simulink library "tqd"  (R2021b)
settings: Solver=VariableStepAuto  StartTime=0.0  StopTime=10.0  RelTol=1e-3
undefined symbols (not defined in the file): ATQD_AfterTqMinGain_X_Deg, ATQD_APSCreepBaseTqD_X_kph, ATQD_APSCreepBaseTqD_Y_Deg, ATQD_APSCreepBaseTqR_X_kph, ATQD_APSCreepBaseTqR_Y_Deg, ATQD_APSCreepIterm_X_kph, ATQD_APSCreepIterm_Y_kph, ATQD_APSCreepPterm_X_kph, ATQD_APSCreepPterm_Y_kph, ATQD_APSDecReq_X_kph, ATQD_APSDecReq_Y_mps2, ATQD_APSDecReqCMD_X_kph, ATQD_APSDecReqTs_X_pct, ATQD_APSDecTimeGain_X_Deg, ATQD_APSDecTimeGain_Y_s, ATQD_APSReqLowSpd_X_Deg, ATQD_AutoHoldReleaseBPS_X_Deg, ATQD_AWDLoadTrqnsGain_X_kg, ATQD_AWDLoadTrqnsGain_Y_pct, ATQD_BOSEnBPSPosn_X_kph, ATQD_BOSMap_X_rpm, ATQD_BOSMap_Y_pct, ATQD_CreepBaseTqD_X_kph, ATQD_CreepBaseTqD_Y_Deg, ATQD_CreepBaseTqR_X_kph, ATQD_CreepBaseTqR_Y_Deg, ATQD_CreepBPSDisPosn_X_Deg, ATQD_CreepBPSDisPosnR_X_Deg, ATQD_CreepBPSEnPosn_X_Deg, ATQD_CreepBPSEnPosnR_X_Deg, ATQD_CreepDeltaTq_X_kph, ATQD_CreepIterm_X_kph, ATQD_CreepIterm_Y_kph, ATQD_CreepItermMaxLimit_X_pct, ATQD_CreepPreloadTime_X_kph, ATQD_CreepPreloadTq_X_kph, ATQD_CreepPreloadTq_Y_s, ATQD_CreepProtTq_X_Deg, ATQD_CreepPterm_X_kph, ATQD_CreepPterm_Y_kph, ATQD_CreepRrTqSpRat_X_rpm, ATQD_CreepRrTqSpRat_Y_Nm, ATQD_CreepTargetSpdD_X_pct, ATQD_CreepTargetSpdR_X_pct, ATQD_ECOTqMapD_X_rpm, ATQD_ECOTqMapD_Y_pct, ATQD_EMTqMapD_X_rpm, ATQD_EMTqMapD_Y_pct, ATQD_EOPDTqMapDCon_X_rpm, ATQD_EOPDTqMapDCon_Y_Deg, ATQD_EscapeModePedTq_X_pct, ATQD_EscapeModePedTq_Y_rpm, ATQD_EscapeModePedTqFr_X_pct, ATQD_EscapeModePedTqFr_Y_rpm, ATQD_EstInitVehWeight_X_c, ATQD_FAfterTqCMDGain_X_rpm, ATQD_FAfterTqCMDGain_Y_pct, ATQD_FrLossMAPLowV_X_rpm, ATQD_FrLossMAPLowV_Y_Nm, ATQD_FrMotActReduce_X_rpm ... (+772)
libraries: simulink x211, hcu_lib x179, tqr x3
(part 5 of 28)

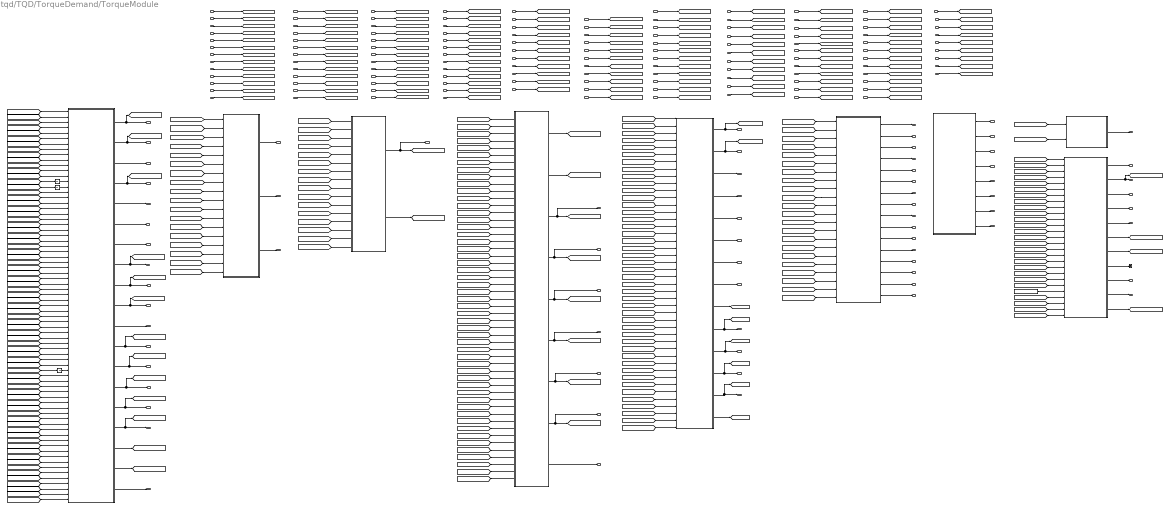
== system tqd/TQD/TorqueDemand/TorqueModule ==
  note: Input Signals
  VTQD_LowIdleAccPedal_flg : Inport
  VPMM_DrivetrainSelect_enum : Inport  Port=2
  VTQD_RollRegenDisableReq_flg : Inport  Port=3
  VTQD_GearActualPosn_enum : Inport  Port=4
  VTQD_CreepON_flg : Inport  Port=5
  VTQD_BrkSwSta_flg : Inport  Port=6
  VTQD_LimpHomeAct_flg : Inport  Port=7
  VTQD_EVDriveMode_enum : Inport  Port=8
  VTQD_RegenMode_enum : Inport  Port=9
  VINP_VehSpeed_kph : Inport  Port=10
  VTQD_TqTargetShaftSpd_rpm : Inport  Port=11
  VTQD_FrShaftSpd_rpm : Inport  Port=12
  VTQD_RrShaftSpd_rpm : Inport  Port=13
  VTQD_ActAPSPosn_pct : Inport  Port=14
  VTQD_ActBPSPosn_pct : Inport  Port=15
  VINP_FrPTCSActive_flg : Inport  Port=16
  VINP_RrPTCSActive_flg : Inport  Port=17
  VINP_FrntAxlTrqReqDrv_Nm : Inport  Port=18
  VINP_RearAxlTrqReqDrv_Nm : Inport  Port=19
  VINP_FrRBCActive_flg : Inport  Port=20
  VINP_RrRBCActive_flg : Inport  Port=21
  VINP_FrntAxlTrqReqBrk_Nm : Inport  Port=22
  VINP_RearAxlTrqReqBrk_Nm : Inport  Port=23
  VVMC_ADASActive_flg : Inport  Port=24
  VVMC_ADASWhlTqReq_Nm : Inport  Port=25
  VVMC_CruzActive_flg : Inport  Port=26
  VVMC_CruzWhlTqReq_Nm : Inport  Port=27
  VVMC_MSAActive_flg : Inport  Port=28
  VVMC_MSAWhlTqReq_Nm : Inport  Port=29
  VVMC_APSActive_flg : Inport  Port=30
  VINP_HVBPwrAvailDchrg_kw : Inport  Port=31
  VTQD_EstVehWeightResult_kg : Inport  Port=32
  VVMC_LongAcc_Gps : Inport  Port=33
  VINP_HVBPwrAvailChrg_kw : Inport  Port=34
  VINP_FrRegenAvailTq_Nm : Inport  Port=35
  VINP_RrRegenAvailTq_Nm : Inport  Port=36
  VINP_FrTMSpd_RPM : Inport  Port=37
  VINP_RrTMSpd_RPM : Inport  Port=38
  VINP_FrEDURealTMTq_Nm : Inport  Port=39
  VINP_RrEDURealTMTq_Nm : Inport  Port=40
  VTQD_ParkRequest_flg : Inport  Port=41
  VPMM_PwrSta_enum : Inport  Port=42
  VTQD_MCUReady4Ext_flg : Inport  Port=43
  VINP_HVBattErr_flg : Inport  Port=44
  VINP_DCDCFaultSta_enum : Inport  Port=45
  VINP_ADASForceIdle_flg : Inport  Port=46
  VTQD_TMRotateDirction_enum : Inport  Port=47
  VINP_LongAccel_Gps : Inport  Port=48
  VTQR_ActualFEDUWhlTqReq_Nm : Inport  Port=49
  VTQR_ActualREDUWhlTqReq_Nm : Inport  Port=50
  VINP_BrkPedalPos_pct : Inport  Port=51
  VTQD_RDCActive_enum : Inport  Port=52
  VVMC_ActMaxSlideRate_pct : Inport  Port=53
  VINP_FrMotorAvailTq_Nm : Inport  Port=54
  VINP_RrMotorAvailTq_Nm : Inport  Port=55
  task_time_s : Inport  Port=56
  VINP_HSAActive_flg : Inport  Port=57
  VTQR_NoABSFEDUWhlTqReq_Nm : Inport  Port=58
  VTQR_NoABSREDUWhlTqReq_Nm : Inport  Port=59
  VINP_AVHActive_flg : Inport  Port=60
  VINP_EPBErrSta_enum : Inport  Port=61
  VVMC_APSSpeedCMD_kph : Inport  Port=62
  VVMC_APSReq_enum : Inport  Port=63
  VINP_ACCVehHoldReq_flg : Inport  Port=64
  VTQD_DriveProtRemove_flg : Inport  Port=65
  VVMC_ACCRequiredAccel_mps2 : Inport  Port=66
  VVMC_EstSlope_Deg : Inport  Port=67
  VTQD_SysMode_enum : Inport  Port=68
  VINP_SWCResUpSta_flg : Inport  Port=69
  VINP_DrDoorSW_flg : Inport  Port=70
  VINP_PsDoorSW_flg : Inport  Port=71
  VINP_RRDoorSW_flg : Inport  Port=72
  VINP_RLDoorSW_flg : Inport  Port=73
  VINP_HoodSW_flg : Inport  Port=74
  VINP_TailgateSW_flg : Inport  Port=75
  VINP_ADASACCSta_enum : Inport  Port=76
  VINP_EPBSta_enum : Inport  Port=77
  VVMC_ActLRSlideRate_pct : Inport  Port=78
  VVMC_ActRRSlideRate_pct : Inport  Port=79
  VINP_SASAngle_Deg : Inport  Port=80
  VINP_YawRate_degps : Inport  Port=81
  VVMC_ActStESCYaw_degps : Inport  Port=82
  VVMC_CAASActive_flg : Inport  Port=83
  VINP_HVBattSOC_pct : Inport  Port=84
  VVMC_RearTqRatio_rat : Inport  Port=85
  VINP_ESCActive_flg : Inport  Port=86
  VINP_ABSActive_flg : Inport  Port=87
  VINP_IVISnowModeCmd_flg : Inport  Port=88
  VINP_VehicleType_enum : Inport  Port=89
  VTQD_IVIRockModeEn_flg : Inport  Port=90
  VTQR_RShaftSpdTqLimLow_flg : Inport  Port=91
  VTQR_RTimerTqLimLow_flg : Inport  Port=92
  VTQR_FShaftSpdTqLimLow_flg : Inport  Port=93
  VTQR_FTimerTqLimLow_flg : Inport  Port=94
  VINP_LFRawWhlSpeed_kph : Inport  Port=95
  VINP_LRRawWhlSpeed_kph : Inport  Port=96
  VINP_RFRawWhlSpeed_kph : Inport  Port=97
  VINP_RRRawWhlSpeed_kph : Inport  Port=98
  VTQD_RearSlideRate_pct : Inport  Port=99
  VTQD_FrontSlideRate_pct : Inport  Port=100
  VINP_SWC2RCustomizeSta_flg : Inport  Port=101
  VTQR_FrFirstOrderInpTs_c : Inport  Port=102
  VTQR_RrFirstOrderInpTs_c : Inport  Port=103
  VTQR_FrRateLimitInc_Nm : Inport  Port=104
  VTQR_FrRateLimitDec_Nm : Inport  Port=105
  VTQR_RrRateLimitInc_Nm : Inport  Port=106
  VTQR_RrRateLimitDec_Nm : Inport  Port=107
  VINP_FrMCUDCBusVolt_V : Inport  Port=108
  VINP_RrMCUDCBusVolt_V : Inport  Port=109
  VTQD_ActWhlSkipSta_enum : Inport  Port=110
  VTQD_SkipDirect_enum : Inport  Port=111
  VDDM_EPB1Err_flg : Inport  Port=112
  VDDM_ESC1Err_flg : Inport  Port=113
  VDDM_ESC5Err_flg : Inport  Port=114
  VDDM_EPBSigErrCFS_flg : Inport  Port=115
  VINP_FrMCUTemp_C : Inport  Port=116
  VINP_FrTMTemp_C : Inport  Port=117
  VINP_RrMCUTemp_C : Inport  Port=118
  VINP_RrTMTemp_C : Inport  Port=119
  VINP_ADASAEBSta_enum : Inport  Port=120
  VTQR_FrTqZeroTransLowBound_Nm : Inport  Port=121
  VTQR_RrTqZeroTransUpBound_Nm : Inport  Port=122
  VDDM_VehMalfunLevel_enum : Inport  Port=123
  VDDM_MCUF1Err_flg : Inport  Port=124
  VDDM_MCUR1Err_flg : Inport  Port=125
  VDDM_Shifter1Err_flg : Inport  Port=126
  VDDM_ShifterSigErrCFS_flg : Inport  Port=127
  VDDM_4D2CErr_flg : Inport  Port=128
  VDDM_RegenErrCFS_flg : Inport  Port=129
  VDDM_VCURAPSErrLv2_flg : Inport  Port=130
  AvaliableTqLimit : Subsystem  AncestorBlock=tqd0/TQD/TorqueDemand/TorqueModule/AvaliableTqLimit
  Constant34 : Constant  Value=KTQD_IVICreepOnSW_flg
  DriverWhlTqDem : Subsystem
  ExtTqFuncHandShaking : Subsystem
  OPD Hold : Subsystem
  Signal for ESC : Subsystem  AncestorBlock=tqd0/TQD/TorqueDemand/TorqueModule/Signal for ESC
  Signals for BCM : Subsystem
  Signals for MCU : Subsystem
  Terminator : Terminator
  TqCoordination : Subsystem
  TqDistribution : Subsystem  AncestorBlock=tqd0/TQD/TorqueDemand/TorqueModule/TqDistribution
  Unit Delay : UnitDelay  SampleTime=-1  HasFrameUpgradeWarning=on
  Unit Delay1 : UnitDelay  SampleTime=-1  HasFrameUpgradeWarning=on
  Unit Delay2 : UnitDelay  SampleTime=-1  HasFrameUpgradeWarning=on
  VTQD_DriverWhlTqDem_Nm : Outport
  VTQD_TqSourceFr_enum : Outport  Port=2
  VTQD_TqSourceRr_enum : Outport  Port=3
  VTQD_RollRegenEnable_flg : Outport  Port=4
  VTQD_EVDriveModeValid_flg : Outport  Port=5
  VTQD_AfterAvailableTqDemFr_Nm : Outport  Port=6
  VTQD_AfterAvailableTqDemRr_Nm : Outport  Port=7
  VTQD_FrEDUAvailBrkRgnTq_Nm : Outport  Port=8
  VTQD_RrEDUAvailBrkRgnTq_Nm : Outport  Port=9
  VTQD_FrRgnDecrSta_flg : Outport  Port=10
  VTQD_RrRgnDecrSta_flg : Outport  Port=11
  VTQD_FrEDUActTq_Nm : Outport  Port=12
  VTQD_RrEDUActTq_Nm : Outport  Port=13
  VTQD_FrEDURolRgnTq_Nm : Outport  Port=14
  VTQD_RrEDURolRgnTq_Nm : Outport  Port=15
  VTQD_FrEDUSpd_rpm : Outport  Port=16
  VTQD_RrEDUSpd_rpm : Outport  Port=17
  VTQD_FrEDUSpdValid_flg : Outport  Port=18
  VTQD_FrEDUActTqValid_flg : Outport  Port=19
  VTQD_FrEDURolRgnTqValid_flg : Outport  Port=20
  VTQD_FrEDUAvailBrkRgnTqV_flg : Outport  Port=21
  VTQD_RrEDUSpdValid_flg : Outport  Port=22
  VTQD_RrEDUActTqValid_flg : Outport  Port=23
  VTQD_RrEDURolRgnTqValid_flg : Outport  Port=24
  VTQD_RrEDUAvailBrkRgnTqV_flg : Outport  Port=25
  VTQD_RgnAbnorSta_flg : Outport  Port=26
  VTQD_PTCSPermSta_flg : Outport  Port=27
  VTQD_FrRgnPermSta_flg : Outport  Port=28
  VTQD_RrRgnPermSta_flg : Outport  Port=29
  VTQD_DriverWhlTqDemFr_Nm : Outport  Port=30
  VTQD_DriverWhlTqDemRr_Nm : Outport  Port=31
  VTQD_ExternalTqAllow_flg : Outport  Port=32
  VTQD_FrIdcMin_A : Outport  Port=33
  VTQD_FrIdcMax_A : Outport  Port=34
  VTQD_FrUdcMin_V : Outport  Port=35
  VTQD_FrUdcMax_V : Outport  Port=36
  VTQD_RrIdcMin_A : Outport  Port=37
  VTQD_RrIdcMax_A : Outport  Port=38
  VTQD_RrUdcMin_V : Outport  Port=39
  VTQD_RrUdcMax_V : Outport  Port=40
  VTQD_CoordWhlTqDemFr_Nm : Outport  Port=41
  VTQD_CoordWhlTqDemRr_Nm : Outport  Port=42
  VTQD_CreepEnable_flg : Outport  Port=43
  VTQD_ReBrakeLPReq_flg : Outport  Port=44
  VTQD_LoSpdBrkCtrl_flg : Outport  Port=45
  VTQD_BOSEnable_flg : Outport  Port=46
  VTQD_ExtShftAllow_flg : Outport  Port=47
  VTQD_OPDOn2Off_flg : Outport  Port=48
  VTQD_PreLoadHold_flg : Outport  Port=49
  VTQD_PreLoadPreEn_flg : Outport  Port=50
  VTQD_CreepPrLoadEnable_flg : Outport  Port=51
  VTQD_APSStaSys_enum : Outport  Port=52
  VTQD_APSReq_enum : Outport  Port=53
  VTQD_APSDecReqA_flg : Outport  Port=54
  VTQD_APSDecReq_mps2 : Outport  Port=55
  VTQD_ActParkRequest_flg : Outport  Port=56
  VTQD_RegenTqLimitEn_flg : Outport  Port=57
  VTQD_ExtDoorAllow_flg : Outport  Port=58
  VTQD_WhlTqCapGenFr_Nm : Outport  Port=59
  VTQD_WhlTqCapGenRr_Nm : Outport  Port=60
  VTQD_OPDHoldAllowPark_flg : Outport  Port=61
  VTQD_OPDHoldLamp_flg : Outport  Port=62
  VTQD_CreepBaseTqD_Nm : Outport  Port=63
  VTQD_VehActSpd_kph : Outport  Port=64
  VTQD_CoordTqDem_Nm : Outport  Port=65
  VTQD_PedAccTqEn_flg : Outport  Port=66
  VTQD_WhlTqCapMotFr_Nm : Outport  Port=67
  VTQD_WhlTqCapMotRr_Nm : Outport  Port=68
  VTQD_CreepTCSActive_flg : Outport  Port=69
  VTQD_EscapModeTqLim_flg : Outport  Port=70
  VTQD_TMEnOutpTqSta_enum : Outport  Port=71
  VTQD_SlideRegenLimTq_Nm : Outport  Port=72
  wires:
  VTQD_ActAPSPosn_pct/1 -> [VTQD_ActAPSPosn_pct]
  VTQD_GearActualPosn_enum/1 -> [VTQD_GearActualPosn_enum]
  VINP_VehSpeed_kph/1 -> [VINP_VehSpeed_kph]
  VTQD_BrkSwSta_flg/1 -> [VTQD_BrkSwSta_flg]
  VTQD_RegenMode_enum/1 -> [VTQD_RegenMode_enum]
  VINP_FrntAxlTrqReqDrv_Nm/1 -> [VINP_FrntAxlTrqReqDrv_Nm]
  VINP_RearAxlTrqReqDrv_Nm/1 -> [VINP_RearAxlTrqReqDrv_Nm]
  VINP_FrPTCSActive_flg/1 -> [VINP_FrPTCSActive_flg]
  VINP_FrntAxlTrqReqBrk_Nm/1 -> [VINP_FrntAxlTrqReqBrk_Nm]
  VINP_RearAxlTrqReqBrk_Nm/1 -> [VINP_RearAxlTrqReqBrk_Nm]
  VTQD_RollRegenDisableReq_flg/1 -> [VTQD_RollRegenDisableReq_flg]
  VINP_FrRBCActive_flg/1 -> [VINP_FrRBCActive_flg]
  VTQD_ActBPSPosn_pct/1 -> [VTQD_ActBPSPosn_pct]
  VVMC_CruzWhlTqReq_Nm/1 -> [VVMC_CruzWhlTqReq_Nm]
  VVMC_CruzActive_flg/1 -> [VVMC_CruzActive_flg]
  VTQD_EVDriveMode_enum/1 -> [VTQD_EVDriveMode_enum]
  VTQD_LimpHomeAct_flg/1 -> [VTQD_LimpHomeAct_flg]
  VTQD_CreepON_flg/1 -> [VTQD_CreepON_flg]
  VTQD_TqTargetShaftSpd_rpm/1 -> [VTQD_TqTargetShaftSpd_rpm]
  VPMM_DrivetrainSelect_enum/1 -> [VPMM_DrivetrainSelect_enum]
  [VTQD_TqTargetShaftSpd_rpm] -> DriverWhlTqDem/10(VTQD_TqTargetShaftSpd_rpm)
  [VTQD_LimpHomeAct_flg] -> DriverWhlTqDem/6(VTQD_LimpHomeAct_flg)
  [VTQD_EVDriveMode_enum] -> DriverWhlTqDem/7(VTQD_EVDriveMode_enum)
  [VTQD_RegenMode_enum] -> DriverWhlTqDem/8(VTQD_RegenMode_enum)
  [VTQD_CreepON_flg] -> DriverWhlTqDem/4("VTQD_CreepON_flg ")
  [VTQD_GearActualPosn_enum] -> DriverWhlTqDem/3(VTQD_GearActualPosn_enum)
  [VTQD_LowIdleAccPedal_flg] -> DriverWhlTqDem/1(VDHP_LowIdleAccPedal_flg)
  [VTQD_ActAPSPosn_pct] -> DriverWhlTqDem/11(VTQD_ActAPSPosn_pct)
  TqDistribution/2(VTQD_RrEDUSpRat_rat) -> [VTQD_RrEDUSpRat_rat]
  TqDistribution/1(VTQD_FrEDUSpRat_rat) -> [VTQD_FrEDUSpRat_rat]
  VINP_HVBPwrAvailChrg_kw/1 -> [VINP_HVBPwrAvailChrg_kw]
  VINP_HVBPwrAvailDchrg_kw/1 -> [VINP_HVBPwrAvailDchrg_kw]
  DriverWhlTqDem/1(VTQD_DriverWhlTqDem_Nm) -> [VTQD_DriverWhlTqDem_Nm], VTQD_DriverWhlTqDem_Nm/1
  [VPMM_DrivetrainSelect_enum] -> TqDistribution/1(VPMM_DrivetrainSelect_enum)
  VVMC_MSAActive_flg/1 -> [VVMC_MSAActive_flg]
  VVMC_MSAWhlTqReq_Nm/1 -> [VVMC_MSAWhlTqReq_Nm]
  VVMC_APSActive_flg/1 -> [VVMC_APSActive_flg]
  VVMC_ADASActive_flg/1 -> [VVMC_ADASActive_flg]
  VVMC_ADASWhlTqReq_Nm/1 -> [VVMC_ADASWhlTqReq_Nm]
  [VTQD_BrkSwSta_flg] -> DriverWhlTqDem/5(VTQD_BrkSwSta_flg)
  [VTQD_ActBPSPosn_pct] -> DriverWhlTqDem/12(VTQD_ActBPSPosn_pct)
  [VINP_VehSpeed_kph] -> DriverWhlTqDem/9(VINP_VehSpeed_kph)
  [VTQD_RollRegenDisableReq_flg] -> DriverWhlTqDem/2(VTQD_RollRegenDisableReq_flg)
  VTQD_FrShaftSpd_rpm/1 -> [VTQD_FrShaftSpd_rpm]
  VTQD_RrShaftSpd_rpm/1 -> [VTQD_RrShaftSpd_rpm]
  VTQD_LowIdleAccPedal_flg/1 -> [VTQD_LowIdleAccPedal_flg]
  DriverWhlTqDem/2(VTQD_RollRegenEnable_flg) -> VTQD_RollRegenEnable_flg/1, [VTQD_RollRegenEnable_flg]
  DriverWhlTqDem/3(VTQD_EVDriveModeValid_flg) -> VTQD_EVDriveModeValid_flg/1
  VINP_RrPTCSActive_flg/1 -> [VINP_RrPTCSActive_flg]
  VINP_RrRBCActive_flg/1 -> [VINP_RrRBCActive_flg]
  VINP_RrTMSpd_RPM/1 -> [VINP_RrTMSpd_rpm]
  VINP_FrTMSpd_RPM/1 -> [VINP_FrTMSpd_rpm]
  VINP_RrRegenAvailTq_Nm/1 -> [VINP_RrRegenAvailTq_Nm]
  VINP_FrRegenAvailTq_Nm/1 -> [VINP_FrRegenAvailTq_Nm]
  VINP_RrEDURealTMTq_Nm/1 -> [VINP_RrEDURealTMTq_Nm]
  VINP_FrEDURealTMTq_Nm/1 -> [VINP_FrEDURealTMTq_Nm]
  AvaliableTqLimit/8(VTQD_RrRgnPermSta_flg) -> VTQD_RrRgnPermSta_flg/1  "VTQD_RrRgnPermSta_flg"
  AvaliableTqLimit/6(VTQD_RrRgnDecrSta_flg) -> VTQD_RrRgnDecrSta_flg/1  "VTQD_RrRgnDecrSta_flg"
  AvaliableTqLimit/7(VTQD_FrRgnPermSta_flg) -> VTQD_FrRgnPermSta_flg/1  "VTQD_FrRgnPermSta_flg"
  [VTQD_RrShaftSpd_rpm] -> AvaliableTqLimit/2(VTQD_RrShaftSpd_rpm)
  [VTQD_FrShaftSpd_rpm] -> AvaliableTqLimit/1(VTQD_FrShaftSpd_rpm)
  AvaliableTqLimit/1(VTQD_AfterAvailableTqDemFr_Nm) -> [VTQD_AfterAvailableTqDemFr_Nm], VTQD_AfterAvailableTqDemFr_Nm/1
  AvaliableTqLimit/5(VTQD_FrRgnDecrSta_flg) -> VTQD_FrRgnDecrSta_flg/1  "VTQD_FrRgnDecrSta_flg"
  AvaliableTqLimit/2(VTQD_AfterAvailableTqDemRr_Nm) -> [VTQD_AfterAvailableTqDemRr_Nm], VTQD_AfterAvailableTqDemRr_Nm/1
  AvaliableTqLimit/3(VTQD_FrEDUAvailBrkRgnTq_Nm) -> VTQD_FrEDUAvailBrkRgnTq_Nm/1
  AvaliableTqLimit/4(VTQD_RrEDUAvailBrkRgnTq_Nm) -> VTQD_RrEDUAvailBrkRgnTq_Nm/1
  [VINP_DCDCFaultSta_enum] -> ExtTqFuncHandShaking/4(VINP_DCDCFaultSta_enum)
  [VINP_HVBattErr_flg] -> ExtTqFuncHandShaking/3(VINP_HVBattErr_flg)
  [VTQD_MCUReady4Ext_flg] -> ExtTqFuncHandShaking/2(VTQD_MCUReady4Ext_flg)
  [VPMM_PwrSta_enum] -> ExtTqFuncHandShaking/1(VPMM_PwrSta_enum)
  VINP_HVBattErr_flg/1 -> [VINP_HVBattErr_flg]
  VINP_ADASForceIdle_flg/1 -> [VINP_ADASForceIdle_flg]
  VTQD_MCUReady4Ext_flg/1 -> [VTQD_MCUReady4Ext_flg]
  VPMM_PwrSta_enum/1 -> [VPMM_PwrSta_enum]
  VINP_DCDCFaultSta_enum/1 -> [VINP_DCDCFaultSta_enum]
  ExtTqFuncHandShaking/1(VTQD_ExternalTqAllow_flg) -> VTQD_ExternalTqAllow_flg/1
  VTQD_TMRotateDirction_enum/1 -> [VTQD_TMRotateDirction_enum]
  [VTQD_TMRotateDirction_enum] -> DriverWhlTqDem/13(VTQD_TMRotateDirction_enum)
  Signals for MCU/8(VTQD_RrUdcMax_V) -> VTQD_RrUdcMax_V/1
  Signals for MCU/5(VTQD_RrIdcMin_A) -> VTQD_RrIdcMin_A/1
  Signals for MCU/3(VTQD_FrUdcMin_V) -> VTQD_FrUdcMin_V/1
  Signals for MCU/2(VTQD_FrIdcMax_A) -> VTQD_FrIdcMax_A/1
  Signals for MCU/7(VTQD_RrUdcMin_V) -> VTQD_RrUdcMin_V/1
  Signals for MCU/6(VTQD_RrIdcMax_A) -> VTQD_RrIdcMax_A/1
  Signals for MCU/4(VTQD_FrUdcMax_V) -> VTQD_FrUdcMax_V/1
  Signals for MCU/1(VTQD_FrIdcMin_A) -> VTQD_FrIdcMin_A/1
  [VTQD_TqSourceFr_enum] -> Unit Delay/1
  [VTQD_TqSourceRr_enum] -> Unit Delay1/1
  Unit Delay/1 -> DriverWhlTqDem/14(VTQD_TqSourceFr_enum)
  Unit Delay1/1 -> DriverWhlTqDem/15(VTQD_TqSourceRr_enum)
  DriverWhlTqDem/4(VTQD_CreepEnable_flg) -> VTQD_CreepEnable_flg/1, [VTQD_CreepEnable_flg]
  VINP_LongAccel_Gps/1 -> [VINP_LongAccel_Gps]
  [VINP_LongAccel_Gps] -> Signals for BCM/2(VINP_LongAccel_Gps)
  Signals for BCM/1(VTQD_ReBrakeLPReq_flg) -> VTQD_ReBrakeLPReq_flg/1
  AvaliableTqLimit/9(VTQD_ARegenActive_flg) -> [VTQD_ARegenActive_flg]
  [VTQD_ARegenActive_flg] -> Signals for BCM/1(VTQD_ARegenActive_flg)
  VTQR_ActualFEDUWhlTqReq_Nm/1 -> [VTQR_ActualFEDUWhlTqReq_Nm]
  VTQR_ActualREDUWhlTqReq_Nm/1 -> [VTQR_ActualREDUWhlTqReq_Nm]
  VINP_BrkPedalPos_pct/1 -> [VINP_BrkPedalPos_pct]
  VTQD_RDCActive_enum/1 -> [VTQD_RDCActive_enum]
  [VTQD_RDCActive_enum] -> DriverWhlTqDem/17(VTQD_RDCActive_enum)
  VVMC_ActMaxSlideRate_pct/1 -> [VVMC_ActMaxSlideRate_pct]
  VINP_RrMotorAvailTq_Nm/1 -> [VINP_RrMotorAvailTq_Nm]
  VINP_FrMotorAvailTq_Nm/1 -> [VINP_FrMotorAvailTq_Nm]
  [VINP_FrEDURealTMTq_Nm] -> Signal for ESC/1(VINP_FrEDURealTMTq_Nm)
  [VINP_RrEDURealTMTq_Nm] -> Signal for ESC/2(VINP_RrEDURealTMTq_Nm)
  [VTQD_RollRegenEnable_flg] -> Signal for ESC/3(VTQD_RollRegenEnable_flg)
  [VVMC_ADASActive_flg] -> TqCoordination/2(VVMC_ADASActive_flg)
  [VINP_ADASForceIdle_flg] -> TqCoordination/10(VINP_ADASForceIdle_flg)
  [VTQD_GearActualPosn_enum] -> TqCoordination/1(VTQD_GearActualPosn_enum)
  [VVMC_MSAWhlTqReq_Nm] -> TqCoordination/7(VVMC_MSAWhlTqReq_Nm)
  [VTQD_DriverWhlTqDem_Nm] -> TqCoordination/9(VTQD_DriverWhlTqDem_Nm)
  [VVMC_CruzActive_flg] -> TqCoordination/4(VVMC_CruzActive_flg)
  [VVMC_APSActive_flg] -> TqCoordination/8(VVMC_APSActive_flg)
  [VVMC_ADASWhlTqReq_Nm] -> TqCoordination/3(VVMC_ADASWhlTqReq_Nm)
  [VVMC_CruzWhlTqReq_Nm] -> TqCoordination/5(VVMC_CruzWhlTqReq_Nm)
  [VVMC_MSAActive_flg] -> TqCoordination/6(VVMC_MSAActive_flg)
  task_time_s/1 -> [task_time_s]
  [task_time_s] -> DriverWhlTqDem/18(task_time_s)
  DriverWhlTqDem/5(VTQD_LoSpdBrkCtrl_flg) -> VTQD_LoSpdBrkCtrl_flg/1
  DriverWhlTqDem/6(VTQD_BOSEnable_flg) -> VTQD_BOSEnable_flg/1
  VINP_HSAActive_flg/1 -> [VINP_HSAActive_flg]
  VTQR_NoABSFEDUWhlTqReq_Nm/1 -> [VTQR_NoABSFEDUWhlTqReq_Nm]
  VTQR_NoABSREDUWhlTqReq_Nm/1 -> [VTQR_NoABSREDUWhlTqReq_Nm]
  VINP_AVHActive_flg/1 -> [VINP_AVHActive_flg]
  VINP_EPBErrSta_enum/1 -> [VINP_EPBErrSta_enum]
  VVMC_APSSpeedCMD_kph/1 -> [VVMC_APSSpeedCMD_kph]
  [VINP_HSAActive_flg] -> DriverWhlTqDem/19(VINP_HSAActive_flg)
  [VINP_RrRBCActive_flg] -> DriverWhlTqDem/20(VINP_RrRBCActive_flg)
  [VINP_FrRBCActive_flg] -> DriverWhlTqDem/21(VINP_FrRBCActive_flg)
  [VVMC_ADASActive_flg] -> DriverWhlTqDem/22(VVMC_ADASActive_flg)
  [VTQD_APSReq_enum] -> DriverWhlTqDem/23(VTQD_APSReq_enum)
  [VINP_AVHActive_flg] -> DriverWhlTqDem/24(VINP_AVHActive_flg)
  [VVMC_APSSpeedCMD_kph] -> DriverWhlTqDem/25(VVMC_APSSpeedCMD_kph)
  [VVMC_APSActive_flg] -> DriverWhlTqDem/26(VVMC_APSActive_flg)
  [VINP_EPBErrSta_enum] -> ExtTqFuncHandShaking/5(VINP_EPBErrSta_enum)
  ExtTqFuncHandShaking/2(VTQD_ExtShftAllow_flg) -> VTQD_ExtShftAllow_flg/1
  [VINP_FrntAxlTrqReqBrk_Nm] -> Signal for ESC/4(VINP_FrntAxlTrqReqBrk_Nm)
  [VINP_RearAxlTrqReqBrk_Nm] -> Signal for ESC/5(VINP_RearAxlTrqReqBrk_Nm)
  [VINP_FrRBCActive_flg] -> Signal for ESC/8(VINP_FrRBCActive_flg)
  [VINP_RrRBCActive_flg] -> Signal for ESC/9(VINP_RrRBCActive_flg)
  [VTQR_ActualREDUWhlTqReq_Nm] -> Signal for ESC/11(VTQR_ActualREDUWhlTqReq_Nm)
  [VTQR_NoABSFEDUWhlTqReq_Nm] -> Signal for ESC/12(VTQR_NoABSFEDUWhlTqReq_Nm)
  [VTQR_NoABSREDUWhlTqReq_Nm] -> Signal for ESC/13(VTQR_NoABSREDUWhlTqReq_Nm)
  [VTQD_DriverWhlTqDem_Nm] -> Signal for ESC/14(VTQD_DriverWhlTqDem_Nm)
  [VINP_FrTMSpd_rpm] -> Signal for ESC/6(VINP_FrTMSpd_rpm)
  [VINP_RrTMSpd_rpm] -> Signal for ESC/7(VINP_RrTMSpd_rpm)
  DriverWhlTqDem/7(VTQD_OPDOn2Off_flg) -> VTQD_OPDOn2Off_flg/1
  [VINP_FrEDURealTMTq_Nm] -> DriverWhlTqDem/27(VINP_FrEDURealTMTq_Nm)
  [VINP_RrEDURealTMTq_Nm] -> DriverWhlTqDem/28(VINP_RrEDURealTMTq_Nm)
  DriverWhlTqDem/9(VTQD_PreLoadPreEn_flg) -> VTQD_PreLoadPreEn_flg/1, [VTQD_PreLoadPreEn_flg]
  DriverWhlTqDem/10(VTQD_CreepPrLoadEnable_flg) -> VTQD_CreepPrLoadEnable_flg/1, [VTQD_CreepPrLoadEnable_flg]
  [VVMC_ADASActive_flg] -> Signal for ESC/15(VVMC_ADASActive_flg)
  VINP_ACCVehHoldReq_flg/1 -> [VINP_ACCVehHoldReq_flg]
  VVMC_APSReq_enum/1 -> [VVMC_APSReq_enum]
  DriverWhlTqDem/8(VTQD_PreLoadHold_flg) -> VTQD_PreLoadHold_flg/1, [VTQD_PreLoadHold_flg]
  [VTQD_PreLoadHold_flg] -> TqCoordination/11(VTQD_PreLoadHold_flg)
  VTQD_DriveProtRemove_flg/1 -> [VTQD_DriveProtRemove_flg]
  VVMC_ACCRequiredAccel_mps2/1 -> [VVMC_ACCRequiredAccel_mps2]
  [VVMC_ACCRequiredAccel_mps2] -> Signal for ESC/16(VVMC_ACCRequiredAccel_mps2)
  VTQD_EstVehWeightResult_kg/1 -> [VTQD_EstVehWeightResult_kg]
  VVMC_LongAcc_Gps/1 -> [VVMC_LongAcc_Gps]
  VTQD_ParkRequest_flg/1 -> [VTQD_ParkRequest_flg]
  [VINP_ACCVehHoldReq_flg] -> DriverWhlTqDem/29(VINP_ACCVehHoldReq_flg)
  [VVMC_APSReq_enum] -> DriverWhlTqDem/30(VVMC_APSReq_enum)
  [VTQD_RrShaftSpd_rpm] -> TqDistribution/2(VTQD_RrShaftSpd_rpm)
  [VTQD_DriverWhlTqDem_Nm] -> TqDistribution/3(VTQD_DriverWhlTqDem_Nm)
  [VTQD_EVDriveMode_enum] -> TqDistribution/4(VTQD_EVDriveMode_enum)
  [VTQD_LimpHomeAct_flg] -> TqDistribution/5(VTQD_LimpHomeAct_flg)
  [VVMC_APSActive_flg] -> TqDistribution/6(VVMC_APSActive_flg)
  [VTQD_CreepPrLoadEnable_flg] -> TqDistribution/7(VTQD_CreepPrLoadEnable_flg)
  [VTQD_EstVehWeightResult_kg] -> TqDistribution/8(VTQD_EstVehWeightResult_kg)
  [VTQD_ActBPSPosn_pct] -> OPD Hold/5(VTQD_ActBPSPosn_pct)
  OPD Hold/3(VTQD_APSDecReqA_flg) -> VTQD_APSDecReqA_flg/1
  OPD Hold/5(VTQD_ActParkRequest_flg) -> VTQD_ActParkRequest_flg/1
  OPD Hold/4(VTQD_APSDecReq_mps2) -> VTQD_APSDecReq_mps2/1
  [VVMC_CruzActive_flg] -> OPD Hold/7(VVMC_CruzActive_flg)
  [VTQD_ParkRequest_flg] -> OPD Hold/8(VTQD_ParkRequest_flg)
  [VVMC_ADASActive_flg] -> OPD Hold/6(VVMC_ADASActive_flg)
  [VTQD_RegenMode_enum] -> OPD Hold/2(VTQD_RegenMode_enum)
  OPD Hold/1(VTQD_APSStaSys_enum) -> VTQD_APSStaSys_enum/1
  [task_time_s] -> OPD Hold/1(task_time_s)
  OPD Hold/2(VTQD_APSReq_enum) -> [VTQD_APSReq_enum], VTQD_APSReq_enum/1
  [VTQD_GearActualPosn_enum] -> OPD Hold/3(VTQD_GearActualPosn_enum)
  [VVMC_ActMaxSlideRate_pct] -> DriverWhlTqDem/16(VVMC_ActMaxSlideRate_pct)
  VVMC_EstSlope_Deg/1 -> [VVMC_EstSlope_Deg]
  [VVMC_LongAcc_Gps] -> DriverWhlTqDem/31(VVMC_LongAcc_Gps)
  DriverWhlTqDem/11(VTQD_RegenTqLimitEn_flg) -> VTQD_RegenTqLimitEn_flg/1
  [VVMC_EstSlope_Deg] -> OPD Hold/9(VVMC_EstSlope_Deg)
  [VVMC_EstSlope_Deg] -> DriverWhlTqDem/32(VVMC_EstSlope_Deg)
  [VTQD_SysMode_enum] -> DriverWhlTqDem/33(VTQD_SysMode_enum)
  [VPMM_PwrSta_enum] -> DriverWhlTqDem/34(VPMM_PwrSta_enum)
  [VINP_SWCResUpSta_flg] -> DriverWhlTqDem/35(VINP_SWCResUpSta_flg)
  [VINP_BrkPedalPos_pct] -> DriverWhlTqDem/36(VINP_BrkPedalPos_pct)
  [VTQR_NoABSFEDUWhlTqReq_Nm] -> DriverWhlTqDem/37(VTQR_NoABSFEDUWhlTqReq_Nm)
  [VTQR_NoABSREDUWhlTqReq_Nm] -> DriverWhlTqDem/38(VTQR_NoABSREDUWhlTqReq_Nm)
  [VTQD_APSReqTimer_s] -> DriverWhlTqDem/39(VTQD_APSReqTimer_s)
  [VINP_FrPTCSActive_flg] -> DriverWhlTqDem/40(VINP_FrPTCSActive_flg)
  [VINP_RrPTCSActive_flg] -> DriverWhlTqDem/41(VINP_RrPTCSActive_flg)
  [VINP_ADASACCSta_enum] -> DriverWhlTqDem/42(VINP_ADASACCSta_enum)
  [VINP_EPBSta_enum] -> DriverWhlTqDem/43(VINP_EPBSta_enum)
  DriverWhlTqDem/12(VTQD_VehActSpd_kph) -> VTQD_VehActSpd_kph/1, [VTQD_VehActSpd_kph]
  [VINP_DrDoorSW_flg] -> ExtTqFuncHandShaking/6(VINP_DrDoorSW_flg)
  [VINP_PsDoorSW_flg] -> ExtTqFuncHandShaking/7(VINP_PsDoorSW_flg)
  [VINP_RRDoorSW_flg] -> ExtTqFuncHandShaking/8(VINP_RRDoorSW_flg)
  [VINP_RLDoorSW_flg] -> ExtTqFuncHandShaking/9(VINP_RLDoorSW_flg)
  [VINP_HoodSW_flg] -> ExtTqFuncHandShaking/10(VINP_HoodSW_flg)
  [VINP_TailgateSW_flg] -> ExtTqFuncHandShaking/11(VINP_TailgateSW_flg)
  ExtTqFuncHandShaking/3(VTQD_ExtDoorAllow_flg) -> VTQD_ExtDoorAllow_flg/1
  TqCoordination/1(VTQD_CoordTqDem_Nm) -> VTQD_CoordTqDem_Nm/1, [VTQD_CoordTqDem_Nm]
  TqCoordination/2(VTQD_TqSource_enum) -> [VTQD_TqSource_enum]
  [VTQD_CoordTqDem_Nm] -> TqDistribution/9(VTQD_CoordTqDem_Nm)
  [VTQD_TqSource_enum] -> TqDistribution/10(VTQD_TqSource_enum)
  [VINP_FrRBCActive_flg] -> TqDistribution/11(VINP_FrRBCActive_flg)
  [VINP_RrRBCActive_flg] -> TqDistribution/12(VINP_RrRBCActive_flg)
  [VTQD_RollRegenEnable_flg] -> TqDistribution/13(VTQD_RollRegenEnable_flg)
  [VINP_FrPTCSActive_flg] -> TqDistribution/14(VINP_FrPTCSActive_flg)
  [VINP_RrPTCSActive_flg] -> TqDistribution/15(VINP_RrPTCSActive_flg)
  [VINP_FrntAxlTrqReqDrv_Nm] -> TqDistribution/16(VINP_FrntAxlTrqReqDrv_Nm)
  [VINP_RearAxlTrqReqDrv_Nm] -> TqDistribution/17(VINP_RearAxlTrqReqDrv_Nm)
  TqDistribution/3(VTQD_CoordWhlTqDemFr_Nm) -> VTQD_CoordWhlTqDemFr_Nm/1, [VTQD_CoordWhlTqDemFr_Nm]
  TqDistribution/4(VTQD_CoordWhlTqDemRr_Nm) -> VTQD_CoordWhlTqDemRr_Nm/1, [VTQD_CoordWhlTqDemRr_Nm]
  TqDistribution/5(VTQD_TqSourceFr_enum) -> VTQD_TqSourceFr_enum/1, [VTQD_TqSourceFr_enum]
  TqDistribution/6(VTQD_TqSourceRr_enum) -> VTQD_TqSourceRr_enum/1, [VTQD_TqSourceRr_enum]
  TqDistribution/7(VTQD_DriverWhlTqDemFr_Nm) -> VTQD_DriverWhlTqDemFr_Nm/1, [VTQD_DriverWhlTqDemFr_Nm]
  TqDistribution/8(VTQD_DriverWhlTqDemRr_Nm) -> VTQD_DriverWhlTqDemRr_Nm/1, [VTQD_DriverWhlTqDemRr_Nm]
  [VTQD_VehActSpd_kph] -> OPD Hold/4(VTQD_VehActSpd_kph)
  [VVMC_LongAcc_Gps] -> OPD Hold/10(VVMC_LongAcc_Gps)
  OPD Hold/6(VTQD_APSReqTimer_s) -> [VTQD_APSReqTimer_s]
  VINP_SWCResUpSta_flg/1 -> [VINP_SWCResUpSta_flg]
  VTQD_SysMode_enum/1 -> [VTQD_SysMode_enum]
  VINP_RLDoorSW_flg/1 -> [VINP_RLDoorSW_flg]
  VINP_HoodSW_flg/1 -> [VINP_HoodSW_flg]
  VINP_TailgateSW_flg/1 -> [VINP_TailgateSW_flg]
  VINP_DrDoorSW_flg/1 -> [VINP_DrDoorSW_flg]
  VINP_PsDoorSW_flg/1 -> [VINP_PsDoorSW_flg]
  VINP_RRDoorSW_flg/1 -> [VINP_RRDoorSW_flg]
  VINP_ADASACCSta_enum/1 -> [VINP_ADASACCSta_enum]
  VINP_EPBSta_enum/1 -> [VINP_EPBSta_enum]
  OPD Hold/7(VTQD_OPDHoldEnRel_flg) -> [VTQD_OPDHoldEnRel_flg]
  [VTQD_OPDHoldEnRel_flg] -> DriverWhlTqDem/44(VTQD_OPDHoldEnRel_flg)
  [VVMC_ActLRSlideRate_pct] -> TqDistribution/18(VVMC_ActLRSlideRate_pct)
  [VVMC_ActRRSlideRate_pct] -> TqDistribution/19(VVMC_ActRRSlideRate_pct)
  VVMC_ActRRSlideRate_pct/1 -> [VVMC_ActRRSlideRate_pct]
  VVMC_ActLRSlideRate_pct/1 -> [VVMC_ActLRSlideRate_pct]
  [VVMC_ActStESCYaw_degps] -> DriverWhlTqDem/47(VVMC_ActStESCYaw_degps)
  [VINP_YawRate_degps] -> DriverWhlTqDem/46(VINP_YawRate_degps)
  [VINP_SASAngle_Deg] -> DriverWhlTqDem/45(VINP_SASAngle_Deg)
  VVMC_ActStESCYaw_degps/1 -> [VVMC_ActStESCYaw_degps]
  VINP_YawRate_degps/1 -> [VINP_YawRate_degps]
  VINP_SASAngle_Deg/1 -> [VINP_SASAngle_Deg]
  [VTQR_NoABSREDUWhlTqReq_Nm] -> OPD Hold/12(VTQR_NoABSREDUWhlTqReq_Nm)
  [VTQR_NoABSFEDUWhlTqReq_Nm] -> OPD Hold/11(VTQR_NoABSFEDUWhlTqReq_Nm)
  [VINP_EPBSta_enum] -> OPD Hold/13(VINP_EPBSta_enum)
  OPD Hold/8(VTQD_OPDHoldDelayForP_flg) -> Terminator/1
  VVMC_CAASActive_flg/1 -> [VVMC_CAASActive_flg]
  [VVMC_CAASActive_flg] -> DriverWhlTqDem/48(VVMC_CAASActive_flg)
  [VPMM_PwrSta_enum] -> OPD Hold/14(VPMM_PwrSta_enum)
  [VTQD_LowIdleAccPedal_flg] -> OPD Hold/15(VTQD_LowIdleAccPedal_flg)
  [VTQD_ActAPSPosn_pct] -> OPD Hold/16(VTQD_ActAPSPosn_pct)
  AvaliableTqLimit/10(VTQD_WhlTqCapGenFr_Nm) -> [VTQD_WhlTqCapGenFr_Nm], VTQD_WhlTqCapGenFr_Nm/1
  AvaliableTqLimit/11(VTQD_WhlTqCapGenRr_Nm) -> [VTQD_WhlTqCapGenRr_Nm], VTQD_WhlTqCapGenRr_Nm/1
  VINP_HVBattSOC_pct/1 -> [VINP_HVBattSOC_pct]
  [VINP_HVBattSOC_pct] -> Signal for ESC/17(VINP_HVBattSOC_pct)
  OPD Hold/9(VTQD_OPDHoldAllowPark_flg) -> VTQD_OPDHoldAllowPark_flg/1
  OPD Hold/10(VTQD_OPDHoldLamp_flg) -> VTQD_OPDHoldLamp_flg/1
  DriverWhlTqDem/13(VTQD_CreepBaseTqD_Nm) -> VTQD_CreepBaseTqD_Nm/1, [VTQD_CreepBaseTqD_Nm]
  [VVMC_ADASWhlTqReq_Nm] -> Unit Delay2/1
  Unit Delay2/1 -> DriverWhlTqDem/49(VVMC_LastADASWhlTqReq_Nm)
  [VTQD_OPDHoldActRelTq_Nm] -> DriverWhlTqDem/50(VTQD_OPDHoldActRelTq_Nm)
  OPD Hold/11(VTQD_OPDHoldActRelTq_Nm) -> [VTQD_OPDHoldActRelTq_Nm]
  [VINP_FrPTCSActive_flg] -> OPD Hold/17(VINP_FrPTCSActive_flg)
  [VINP_RrPTCSActive_flg] -> OPD Hold/18(VINP_RrPTCSActive_flg)
  [VINP_ESCActive_flg] -> OPD Hold/19(VINP_ESCActive_flg)
  [VINP_ABSActive_flg] -> OPD Hold/20(VINP_ABSActive_flg)
  VINP_ESCActive_flg/1 -> [VINP_ESCActive_flg]
  VINP_ABSActive_flg/1 -> [VINP_ABSActive_flg]
  [VVMC_APSActive_flg] -> OPD Hold/21(VVMC_APSActive_flg)
  [VINP_IVISnowModeCmd_flg] -> DriverWhlTqDem/51(VINP_IVISnowModeCmd_flg)
  VINP_IVISnowModeCmd_flg/1 -> [VINP_IVISnowModeCmd_flg]
  VINP_VehicleType_enum/1 -> [VINP_VehicleType_enum]
  [VTQD_IVIRockModeEn_flg] -> DriverWhlTqDem/52(VTQD_IVIRockModeEn_flg)
  VTQD_IVIRockModeEn_flg/1 -> [VTQD_IVIRockModeEn_flg]
  [VTQR_RShaftSpdTqLimLow_flg] -> DriverWhlTqDem/53(VTQR_RShaftSpdTqLimLow_flg)
  [VTQR_RTimerTqLimLow_flg] -> DriverWhlTqDem/54(VTQR_RTimerTqLimLow_flg)
  [VTQR_FShaftSpdTqLimLow_flg] -> DriverWhlTqDem/55(VTQR_FShaftSpdTqLimLow_flg)
  [VTQR_FTimerTqLimLow_flg] -> DriverWhlTqDem/56(VTQR_FTimerTqLimLow_flg)
  [VINP_LFRawWhlSpeed_kph] -> DriverWhlTqDem/57(VINP_LFRawWhlSpeed_kph)
  [VINP_LRRawWhlSpeed_kph] -> DriverWhlTqDem/58(VINP_LRRawWhlSpeed_kph)
  [VINP_RFRawWhlSpeed_kph] -> DriverWhlTqDem/59(VINP_RFRawWhlSpeed_kph)
  [VINP_RRRawWhlSpeed_kph] -> DriverWhlTqDem/60(VINP_RRRawWhlSpeed_kph)
  [VTQD_FrShaftSpd_rpm] -> DriverWhlTqDem/61(VTQD_FrShaftSpd_rpm)
  [VTQD_RrShaftSpd_rpm] -> DriverWhlTqDem/62(VTQD_RrShaftSpd_rpm)
  VTQR_FTimerTqLimLow_flg/1 -> [VTQR_FTimerTqLimLow_flg]
  VTQR_FShaftSpdTqLimLow_flg/1 -> [VTQR_FShaftSpdTqLimLow_flg]
  VTQR_RTimerTqLimLow_flg/1 -> [VTQR_RTimerTqLimLow_flg]
  VTQR_RShaftSpdTqLimLow_flg/1 -> [VTQR_RShaftSpdTqLimLow_flg]
  VINP_RRRawWhlSpeed_kph/1 -> [VINP_RRRawWhlSpeed_kph]
  VINP_RFRawWhlSpeed_kph/1 -> [VINP_RFRawWhlSpeed_kph]
  VINP_LRRawWhlSpeed_kph/1 -> [VINP_LRRawWhlSpeed_kph]
  VINP_LFRawWhlSpeed_kph/1 -> [VINP_LFRawWhlSpeed_kph]
  DriverWhlTqDem/14(VTQD_PedAccTqEn_flg) -> VTQD_PedAccTqEn_flg/1, [VTQD_PedAccTqEn_flg]
  DriverWhlTqDem/15(VTQD_EscapModeTqLim_flg) -> VTQD_EscapModeTqLim_flg/1, [VTQD_EscapModeTqLim_flg]
  VVMC_RearTqRatio_rat/1 -> [VVMC_RearTqRatio_rat]
  [VVMC_RearTqRatio_rat] -> TqDistribution/20(VVMC_RearTqRatio_rat)
  [VTQD_FrontSlideRate_pct] -> TqDistribution/21(VTQD_FrontSlideRate_pct)
  [VTQD_RearSlideRate_pct] -> TqDistribution/22(VTQD_RearSlideRate_pct)
  VTQD_RearSlideRate_pct/1 -> [VTQD_RearSlideRate_pct]
  VTQD_FrontSlideRate_pct/1 -> [VTQD_FrontSlideRate_pct]
  [VINP_HVBPwrAvailDchrg_kw] -> AvaliableTqLimit/3(VINP_HVBPwrAvailDchrg_kw)
  [VINP_HVBPwrAvailChrg_kw] -> AvaliableTqLimit/4(VINP_HVBPwrAvailChrg_kw)
  [VTQD_CoordWhlTqDemFr_Nm] -> AvaliableTqLimit/5(VTQD_CoordWhlTqDemFr_Nm)
  [VTQD_CoordWhlTqDemRr_Nm] -> AvaliableTqLimit/6(VTQD_CoordWhlTqDemRr_Nm)
  [VTQD_FrEDUSpRat_rat] -> AvaliableTqLimit/7(VTQD_FrEDUSpRat_rat)
  [VTQD_RrEDUSpRat_rat] -> AvaliableTqLimit/8(VTQD_RrEDUSpRat_rat)
  [VTQD_TqSourceFr_enum] -> AvaliableTqLimit/9(VTQD_TqSourceFr_enum)
  [VTQD_TqSourceRr_enum] -> AvaliableTqLimit/10(VTQD_TqSourceRr_enum)
  [VTQD_DriverWhlTqDemFr_Nm] -> AvaliableTqLimit/11(VTQD_DriverWhlTqDemFr_Nm)
  [VTQD_DriverWhlTqDemRr_Nm] -> AvaliableTqLimit/12(VTQD_DriverWhlTqDemRr_Nm)
  [VINP_FrRegenAvailTq_Nm] -> AvaliableTqLimit/13(VINP_FrRegenAvailTq_Nm)
  [VINP_RrRegenAvailTq_Nm] -> AvaliableTqLimit/14(VINP_RrRegenAvailTq_Nm)
  [VTQD_DriverWhlTqDem_Nm] -> AvaliableTqLimit/15(VTQD_DriverWhlTqDem_Nm)
  [VINP_FrMotorAvailTq_Nm] -> AvaliableTqLimit/16(VINP_FrMotorAvailTq_Nm)
  [VINP_RrMotorAvailTq_Nm] -> AvaliableTqLimit/17(VINP_RrMotorAvailTq_Nm)
  [VTQD_CreepEnable_flg] -> AvaliableTqLimit/18(VTQD_CreepEnable_flg)
  [VVMC_ADASActive_flg] -> AvaliableTqLimit/19(VVMC_ADASActive_flg)
  [VTQD_DriveProtRemove_flg] -> AvaliableTqLimit/20(VTQD_DriveProtRemove_flg)
  [VINP_FrPTCSActive_flg] -> AvaliableTqLimit/21(VINP_FrPTCSActive_flg)
  [VINP_RrPTCSActive_flg] -> AvaliableTqLimit/22(VINP_RrPTCSActive_flg)
  [VINP_FrntAxlTrqReqDrv_Nm] -> AvaliableTqLimit/23(VINP_FrntAxlTrqReqDrv_Nm)
  [VINP_RearAxlTrqReqDrv_Nm] -> AvaliableTqLimit/24(VINP_RearAxlTrqReqDrv_Nm)
  [VTQD_VehActSpd_kph] -> AvaliableTqLimit/25(VTQD_VehActSpd_kph)
  [VINP_VehicleType_enum] -> AvaliableTqLimit/36(VINP_VehicleType_enum)
  [VINP_HVBattSOC_pct] -> AvaliableTqLimit/34(VINP_HVBattSOC_pct)
  [VVMC_CAASActive_flg] -> AvaliableTqLimit/27(VVMC_CAASActive_flg)
  [VPMM_DrivetrainSelect_enum] -> AvaliableTqLimit/35(VPMM_DrivetrainSelect_enum)
  [task_time_s] -> AvaliableTqLimit/33(task_time_s)
  [VTQD_IVIRockModeEn_flg] -> AvaliableTqLimit/32(VTQD_IVIRockModeEn_flg)
  [VINP_IVISnowModeCmd_flg] -> AvaliableTqLimit/31(VINP_IVISnowModeCmd_flg)
  [VTQD_RearSlideRate_pct] -> AvaliableTqLimit/30(VTQD_RearSlideRate_pct)
  [VTQD_FrontSlideRate_pct] -> AvaliableTqLimit/29(VTQD_FrontSlideRate_pct)
  [VTQD_GearActualPosn_enum] -> AvaliableTqLimit/28(VTQD_GearActualPosn_enum)
  [VTQD_PreLoadPreEn_flg] -> AvaliableTqLimit/26(VTQD_PreLoadPreEn_flg)
  AvaliableTqLimit/12(VTQD_WhlTqCapMotFr_Nm) -> [VTQD_WhlTqCapMotFr_Nm], VTQD_WhlTqCapMotFr_Nm/1
  AvaliableTqLimit/13(VTQD_WhlTqCapMotRr_Nm) -> [VTQD_WhlTqCapMotRr_Nm], VTQD_WhlTqCapMotRr_Nm/1
  [VTQR_ActualFEDUWhlTqReq_Nm] -> Signal for ESC/10(VTQR_ActualFEDUWhlTqReq_Nm)
  [VTQD_AfterAvailableTqDemFr_Nm] -> Signal for ESC/18(VTQD_AfterAvailableTqDemFr_Nm)
  [VTQD_AfterAvailableTqDemRr_Nm] -> Signal for ESC/19(VTQD_AfterAvailableTqDemRr_Nm)
  [VTQD_GearActualPosn_enum] -> Signal for ESC/20(VTQD_GearActualPosn_enum)
  Signal for ESC/1(VTQD_FrEDUActTq_Nm) -> VTQD_FrEDUActTq_Nm/1
  Signal for ESC/2(VTQD_RrEDUActTq_Nm) -> VTQD_RrEDUActTq_Nm/1
  Signal for ESC/3(VTQD_FrEDURolRgnTq_Nm) -> VTQD_FrEDURolRgnTq_Nm/1
  Signal for ESC/4(VTQD_RrEDURolRgnTq_Nm) -> VTQD_RrEDURolRgnTq_Nm/1
  Signal for ESC/16(VTQD_PTCSPermSta_flg) -> VTQD_PTCSPermSta_flg/1
  Signal for ESC/15(VTQD_RgnAbnorSta_flg) -> VTQD_RgnAbnorSta_flg/1
  Signal for ESC/14(VTQD_RrEDUAvailBrkRgnTqV_flg) -> VTQD_RrEDUAvailBrkRgnTqV_flg/1  "VTQD_RrEDUAvailBrkRgnTqV_flg"
  Signal for ESC/13(VTQD_RrEDURolRgnTqValid_flg) -> VTQD_RrEDURolRgnTqValid_flg/1  "VTQD_RrEDURolRgnTqValid_flg"
  Signal for ESC/12(VTQD_RrEDUActTqValid_flg) -> VTQD_RrEDUActTqValid_flg/1  "VTQD_RrEDUActTqValid_flg"
  Signal for ESC/11(VTQD_RrEDUSpdValid_flg) -> VTQD_RrEDUSpdValid_flg/1  "VTQD_RrEDUSpdValid_flg"
  Signal for ESC/10(VTQD_FrEDUAvailBrkRgnTqV_flg) -> VTQD_FrEDUAvailBrkRgnTqV_flg/1  "VTQD_FrEDUAvailBrkRgnTqV_flg"
  Signal for ESC/9(VTQD_FrEDURolRgnTqValid_flg) -> VTQD_FrEDURolRgnTqValid_flg/1  "VTQD_FrEDURolRgnTqValid_flg"
  Signal for ESC/8(VTQD_FrEDUActTqValid_flg) -> VTQD_FrEDUActTqValid_flg/1  "VTQD_FrEDUActTqValid_flg"
  Signal for ESC/7(VTQD_FrEDUSpdValid_flg) -> VTQD_FrEDUSpdValid_flg/1  "VTQD_FrEDUSpdValid_flg"
  Signal for ESC/6(VTQD_RrEDUSpd_rpm) -> VTQD_RrEDUSpd_rpm/1
  Signal for ESC/5(VTQD_FrEDUSpd_rpm) -> VTQD_FrEDUSpd_rpm/1
  [VTQD_PedAccTqEn_flg] -> OPD Hold/22(VTQD_PedAccTqEn_flg)
  Constant34/1 -> OPD Hold/23(VINP_IVICreepOnSW_flg)  "VTQD_IVICreepOnSW_flg"
  VINP_SWC2RCustomizeSta_flg/1 -> [VINP_SWC2RCustomizeSta_flg]
  [VINP_SWC2RCustomizeSta_flg] -> DriverWhlTqDem/63(VINP_SWC2RCustomizeSta_flg)
  VTQR_RrRateLimitInc_Nm/1 -> [VTQR_RrRateLimitInc_Nm]
  VTQR_RrRateLimitDec_Nm/1 -> [VTQR_RrRateLimitDec_Nm]
  VTQR_FrRateLimitInc_Nm/1 -> [VTQR_FrRateLimitInc_Nm]
  VTQR_FrRateLimitDec_Nm/1 -> [VTQR_FrRateLimitDec_Nm]
  VTQR_FrFirstOrderInpTs_c/1 -> [VTQR_FrFirstOrderInpTs_c]
  VTQR_RrFirstOrderInpTs_c/1 -> [VTQR_RrFirstOrderInpTs_c]
  [VTQR_FrFirstOrderInpTs_c] -> TqDistribution/23(VTQR_FrFirstOrderInpTs_c)
  [VTQR_RrFirstOrderInpTs_c] -> TqDistribution/24(VTQR_RrFirstOrderInpTs_c)
  [VTQR_FrRateLimitInc_Nm] -> TqDistribution/25(VTQR_FrRateLimitInc_Nm)
  [VTQR_FrRateLimitDec_Nm] -> TqDistribution/26(VTQR_FrRateLimitDec_Nm)
  [VTQR_RrRateLimitInc_Nm] -> TqDistribution/27(VTQR_RrRateLimitInc_Nm)
  [VTQR_RrRateLimitDec_Nm] -> TqDistribution/28(VTQR_RrRateLimitDec_Nm)
  [task_time_s] -> TqDistribution/29(task_time_s)
  [VTQD_WhlTqCapMotRr_Nm] -> TqDistribution/33(VTQD_WhlTqCapMotRr_Nm)
  [VTQD_WhlTqCapGenFr_Nm] -> TqDistribution/30(VTQD_WhlTqCapGenFr_Nm)
  [VTQD_WhlTqCapGenRr_Nm] -> TqDistribution/31(VTQD_WhlTqCapGenRr_Nm)
  [VTQD_WhlTqCapMotFr_Nm] -> TqDistribution/32(VTQD_WhlTqCapMotFr_Nm)
  DriverWhlTqDem/16(VTQD_CreepTCSActive_flg) -> VTQD_CreepTCSActive_flg/1, [VTQD_CreepTCSActive_flg]
  [VTQD_CreepBaseTqD_Nm] -> TqDistribution/34(VTQD_CreepBaseTqD_Nm)
  [VTQD_CreepTCSActive_flg] -> TqDistribution/35(VTQD_CreepTCSActive_flg)
  [VTQD_IVIRockModeEn_flg] -> OPD Hold/24(VTQD_IVIRockModeEn_flg)
  [VTQD_EscapModeTqLim_flg] -> TqDistribution/36(VTQD_EscapModeTqLim_flg)
  [VTQD_FrShaftSpd_rpm] -> TqDistribution/37(VTQD_FrShaftSpd_rpm)
  [VTQD_ActAPSPosn_pct] -> TqDistribution/38(VTQD_ActAPSPosn_pct)
  [VTQD_CreepEnable_flg] -> TqDistribution/39(VTQD_CreepEnable_flg)
  [VVMC_EstSlope_Deg] -> AvaliableTqLimit/37(VVMC_EstSlope_Deg)
  [VINP_FrMCUDCBusVolt_V] -> AvaliableTqLimit/38(VINP_FrMCUDCBusVolt_V)
  [VINP_RrMCUDCBusVolt_V] -> AvaliableTqLimit/39(VINP_RrMCUDCBusVolt_V)
  VINP_FrMCUDCBusVolt_V/1 -> [VINP_FrMCUDCBusVolt_V]
  VINP_RrMCUDCBusVolt_V/1 -> [VINP_RrMCUDCBusVolt_V]
  VTQD_ActWhlSkipSta_enum/1 -> [VTQD_ActWhlSkipSta_enum]
  VTQD_SkipDirect_enum/1 -> [VTQD_SkipDirect_enum]
  [VTQD_ActWhlSkipSta_enum] -> DriverWhlTqDem/64(VTQD_ActWhlSkipSta_enum)
  [VTQD_ActWhlSkipSta_enum] -> OPD Hold/25(VTQD_ActWhlSkipSta_enum)
  [VTQD_SkipDirect_enum] -> OPD Hold/26(VTQD_SkipDirect_enum)
  VDDM_EPB1Err_flg/1 -> [VDDM_EPB1Err_flg]
  VDDM_ESC5Err_flg/1 -> [VDDM_ESC5Err_flg]
  VDDM_ESC1Err_flg/1 -> [VDDM_ESC1Err_flg]
  VDDM_EPBSigErrCFS_flg/1 -> [VDDM_EPBSigErrCFS_flg]
  [VDDM_EPBSigErrCFS_flg] -> DriverWhlTqDem/68(VDDM_EPBSigErrCFS_flg)
  [VDDM_ESC5Err_flg] -> DriverWhlTqDem/67(VDDM_ESC5Err_flg)
  [VDDM_ESC1Err_flg] -> DriverWhlTqDem/66(VDDM_ESC1Err_flg)
  [VDDM_EPB1Err_flg] -> DriverWhlTqDem/65(VDDM_EPB1Err_flg)
  VINP_FrMCUTemp_C/1 -> [VINP_FrMCUTemp_C]
  VINP_FrTMTemp_C/1 -> [VINP_FrTMTemp_C]
  VINP_RrMCUTemp_C/1 -> [VINP_RrMCUTemp_C]
  VINP_RrTMTemp_C/1 -> [VINP_RrTMTemp_C]
  [VINP_RrTMTemp_C] -> AvaliableTqLimit/43(VINP_RrTMTemp_C)
  [VINP_RrMCUTemp_C] -> AvaliableTqLimit/42(VINP_RrMCUTemp_C)
  [VINP_FrTMTemp_C] -> AvaliableTqLimit/41(VINP_FrTMTemp_C)
  [VINP_FrMCUTemp_C] -> AvaliableTqLimit/40(VINP_FrMCUTemp_C)
  VINP_ADASAEBSta_enum/1 -> [VINP_ADASAEBSta_enum]
  [VINP_ADASAEBSta_enum] -> DriverWhlTqDem/69(VINP_ADASAEBSta_enum)
  [VTQD_ActAPSPosn_pct] -> AvaliableTqLimit/44(VTQD_ActAPSPosn_pct)
  DriverWhlTqDem/18(VTQD_RrPreloadTq_Nm) -> [VTQD_RrPreloadTq_Nm]
  DriverWhlTqDem/17(VTQD_FrPreloadTq_Nm) -> [VTQD_FrPreloadTq_Nm]
  [VTQR_NoABSFEDUWhlTqReq_Nm] -> TqDistribution/40(VTQR_NoABSFEDUWhlTqReq_Nm)
  [VTQR_FrTqZeroTransLowBound_Nm] -> TqDistribution/41(VTQR_FrTqZeroTransLowBound_Nm)
  [VTQR_NoABSREDUWhlTqReq_Nm] -> TqDistribution/42(VTQR_NoABSREDUWhlTqReq_Nm)
  [VTQR_RrTqZeroTransUpBound_Nm] -> TqDistribution/43(VTQR_RrTqZeroTransUpBound_Nm)
  [VINP_RrMotorAvailTq_Nm] -> TqDistribution/44(VINP_RrMotorAvailTq_Nm)
  [VINP_RrRegenAvailTq_Nm] -> TqDistribution/45(VINP_RrRegenAvailTq_Nm)
  [VINP_FrMotorAvailTq_Nm] -> TqDistribution/46(VINP_FrMotorAvailTq_Nm)
  [VINP_FrRegenAvailTq_Nm] -> TqDistribution/47(VINP_FrRegenAvailTq_Nm)
  [VTQD_RrPreloadTq_Nm] -> TqDistribution/48(VTQD_RrPreloadTq_Nm)
  [VTQD_FrPreloadTq_Nm] -> TqDistribution/49(VTQD_FrPreloadTq_Nm)
  [VTQD_PreLoadHold_flg] -> TqDistribution/50(VTQD_PreLoadHold_flg)
  VTQR_FrTqZeroTransLowBound_Nm/1 -> [VTQR_FrTqZeroTransLowBound_Nm]
  VTQR_RrTqZeroTransUpBound_Nm/1 -> [VTQR_RrTqZeroTransUpBound_Nm]
  TqDistribution/9(VTQD_TMEnOutpTqSta_enum) -> VTQD_TMEnOutpTqSta_enum/1
  [VINP_HVBPwrAvailDchrg_kw] -> TqCoordination/12(VINP_HVBPwrAvailDchrg_kW)
  [VINP_HVBPwrAvailChrg_kw] -> TqCoordination/13(VINP_HVBPwrAvailChrg_kW)
  [VTQD_MotorLossTotal_kw] -> TqCoordination/14(VTQD_MotorLossTotal_kw)
  [VTQD_FrShaftSpd_rpm] -> TqCoordination/15(VTQD_FrShaftSpd_rpm)
  [VTQD_RrShaftSpd_rpm] -> TqCoordination/16(VTQD_RrShaftSpd_rpm)
  AvaliableTqLimit/14(VTQD_MotorLossTotal_kw) -> [VTQD_MotorLossTotal_kw]
  VDDM_VehMalfunLevel_enum/1 -> [VDDM_VehMalfunLevel_enum]
  VDDM_MCUR1Err_flg/1 -> [VDDM_MCUR1Err_flg]
  VDDM_MCUF1Err_flg/1 -> [VDDM_MCUF1Err_flg]
  VDDM_RegenErrCFS_flg/1 -> [VDDM_RegenErrCFS_flg]
  VDDM_ShifterSigErrCFS_flg/1 -> [VDDM_ShifterSigErrCFS_flg]
  VDDM_Shifter1Err_flg/1 -> [VDDM_Shifter1Err_flg]
  VDDM_4D2CErr_flg/1 -> [VDDM_4D2CErr_flg]
  [VDDM_VehMalfunLevel_enum] -> DriverWhlTqDem/70(VDDM_VehMalfunLevel_enum)
  [VDDM_MCUF1Err_flg] -> DriverWhlTqDem/71(VDDM_MCUF1Err_flg)
  [VDDM_MCUR1Err_flg] -> DriverWhlTqDem/72(VDDM_MCUR1Err_flg)
  [VDDM_Shifter1Err_flg] -> ExtTqFuncHandShaking/12(VDDM_Shifter1Err_flg)
  [VDDM_ShifterSigErrCFS_flg] -> ExtTqFuncHandShaking/13(VDDM_ShifterSigErrCFS_flg)
  [VTQD_LimpHomeAct_flg] -> ExtTqFuncHandShaking/14(VTQD_LimpHomeAct_flg)
  [VDDM_EPBSigErrCFS_flg] -> ExtTqFuncHandShaking/15(VDDM_EPBSigErrCFS_flg)
  [VDDM_4D2CErr_flg] -> ExtTqFuncHandShaking/16(VDDM_4D2CErr_flg)
  [VDDM_EPB1Err_flg] -> ExtTqFuncHandShaking/17(VDDM_EPB1Err_flg)
  [VPMM_DrivetrainSelect_enum] -> Signal for ESC/21(VPMM_DrivetrainSelect_enum)
  [VDDM_RegenErrCFS_flg] -> Signal for ESC/22(VDDM_RegenErrCFS_flg)
  [VTQD_LimpHomeAct_flg] -> OPD Hold/27(VTQD_LimpHomeAct_flg)
  [VVMC_APSActive_flg] -> ExtTqFuncHandShaking/18(VVMC_APSActive_flg)
  DriverWhlTqDem/19(VTQD_SlideRegenLimTq_Nm) -> VTQD_SlideRegenLimTq_Nm/1
  [VDDM_VCURAPSErrLv2_flg] -> DriverWhlTqDem/73(VDDM_VCURAPSErrLv2_flg)
  VDDM_VCURAPSErrLv2_flg/1 -> [VDDM_VCURAPSErrLv2_flg]
  [VINP_IVISnowModeCmd_flg] -> TqDistribution/51(VINP_IVISnowModeCmd_flg)
